simulink library "lateralFlightController"  (R2018b)
settings: Solver=VariableStepAuto  StartTime=0.0  StopTime=10.0  RelTol=1e-3
values from neighbouring files (symbols this model uses):
  kdRollMom = 5000*(pi/180)*MOI_X    [lateralFlight_ts.m]
  kdVelAng = 6*kpVelAng    (= 48)    [lateralFlight_ts.m]
  kpRollMom = 25000*(pi/180)*MOI_X    [lateralFlight_ts.m]
  kpVelAng = maxBank/(5*(pi/180))    (= 8)    [lateralFlight_ts.m]
  maxBank = 40*pi/180    (= 0.698131700798)    [lateralFlight_ts.m]
  tauRollMom = .01    (= 0.01)    [lateralFlight_ts.m]
  tauVelAng = .01    (= 0.01)    [lateralFlight_ts.m]
libraries: setpointToOutput_cl x2, filteredPIDController_ul x2, cartToSphere_ul x1, vrlib x1, schmehlTangentRotation_ul x1
settings Model: Creator=James Reed  LastModifiedBy=jldanie5

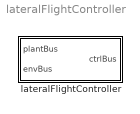
== system lateralFlightController ==
  lateralFlightController : Subsystem

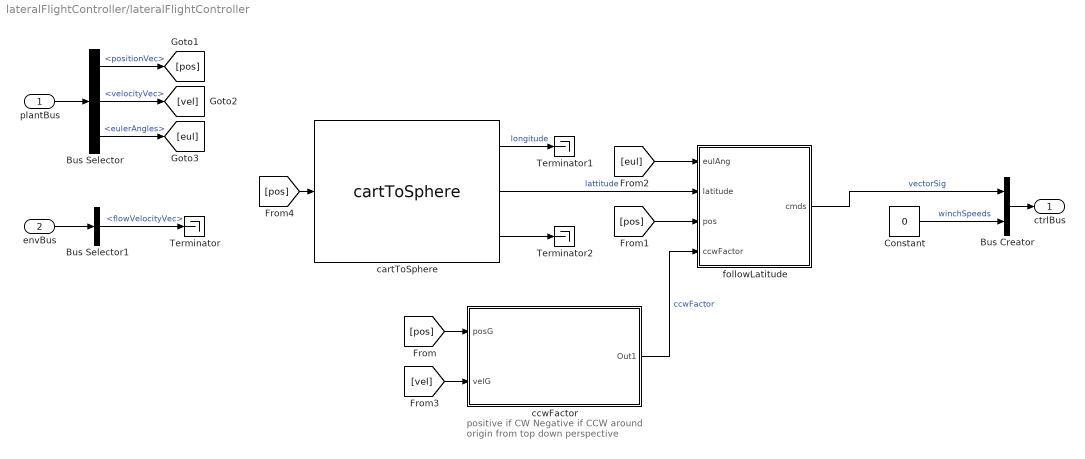
== system lateralFlightController/lateralFlightController ==
  note: positive if CW
      | Negative if CCW
      | around origin from top down perspective
  plantBus : Inport  OutDataTypeStr=Bus: plantBus
  envBus : Inport  Port=2  OutDataTypeStr=Bus: envBus
  Bus Creator : BusCreator  Inputs=2  OutDataTypeStr=Bus: ctrlBus
  Bus Selector : BusSelector  OutputSignals=positionVec,velocityVec,eulerAngles
  Bus Selector1 : BusSelector  OutputSignals=flowVelocityVec
  Constant : Constant  Value=0
  Terminator : Terminator
  Terminator1 : Terminator
  Terminator2 : Terminator
  cartToSphere : cartToSphere_ul/cartToSphere  SystemSampleTime=-1
  ccwFactor : Subsystem
  followLatitude : Subsystem  mask{kpVelAngMask=kpVelAng, kdVelAngMask=kdVelAng, tauVelAngMask=tauVelAng, kpLMask=kpRollMom, kdLMask=kdRollMom, tauLMask=tauRollMom, maxBankMask=maxBank, latDes=pi/4}
      mask prompts: kpVelAngMask "Proportional Gain Velocity Angle"; kdVelAngMask "Derivative Gain Velocity Angle"; tauVelAngMask "Tau Velocity Angle"; kpLMask "Proportional Gain TanRoll"; kdLMask "Derivative Gain Tanroll"; tauLMask "Tau Roll Moment"; maxBankMask "Max Bank Angle"; latDes "Desired Latitude"
  ctrlBus : Outport  OutDataTypeStr=Bus: ctrlBus
  wires:
  Bus Selector/3 -> [eul]  "<eulerAngles>"
  Bus Selector/1 -> [pos]  "<positionVec>"
  Bus Selector1/1 -> Terminator/1  "<flowVelocityVec>"
  Bus Selector/2 -> [vel]  "<velocityVec>"
  plantBus/1 -> Bus Selector/1
  envBus/1 -> Bus Selector1/1
  Bus Creator/1 -> ctrlBus/1
  followLatitude/1(cmds) -> Bus Creator/1  "vectorSig"
  Constant/1 -> Bus Creator/2  "winchSpeeds"
  [eul] -> followLatitude/1(eulAng)
  [pos] -> cartToSphere/1
  cartToSphere/1 -> Terminator1/1  "longitude"
  cartToSphere/3 -> Terminator2/1
  cartToSphere/2 -> followLatitude/2("latitude ")  "lattitude"
  [pos] -> followLatitude/3("pos ")
  [pos] -> ccwFactor/1(posG)
  [vel] -> ccwFactor/2(velG)
  ccwFactor/1(Out1) -> followLatitude/4(ccwFactor)  "ccwFactor"

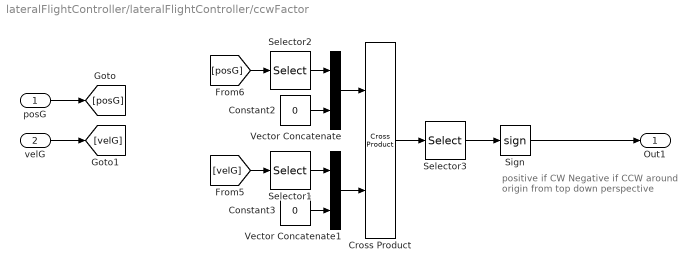
== system lateralFlightController/lateralFlightController/ccwFactor ==
  note: positive if CW
      | Negative if CCW
      | around origin from top down perspective
  posG : Inport
  velG : Inport  Port=2
  Constant2 : Constant  Value=0
  Constant3 : Constant  Value=0
  Cross Product : vrlib/Utilities/Cross Product
      settings: SourceProductBaseCode=VR
  Selector1 : Selector  InputPortWidth=3  IndexOptions=Index vector (dialog)  Indices=[1 2]  OutputSizes=1
  Selector2 : Selector  InputPortWidth=3  IndexOptions=Index vector (dialog)  Indices=[1 2]  OutputSizes=1
  Selector3 : Selector  InputPortWidth=3  IndexOptions=Index vector (dialog)  Indices=3  OutputSizes=1
  Sign : Signum
  Vector Concatenate : Concatenate
  Vector Concatenate1 : Concatenate
  Out1 : Outport
  wires:
  Sign/1 -> Out1/1
  Vector Concatenate1/1 -> Cross Product/2
  Vector Concatenate/1 -> Cross Product/1
  [posG] -> Selector2/1
  Selector1/1 -> Vector Concatenate1/1
  [velG] -> Selector1/1
  Selector2/1 -> Vector Concatenate/1
  Constant2/1 -> Vector Concatenate/2
  Constant3/1 -> Vector Concatenate1/2
  Selector3/1 -> Sign/1
  Cross Product/1 -> Selector3/1
  posG/1 -> [posG]
  velG/1 -> [velG]

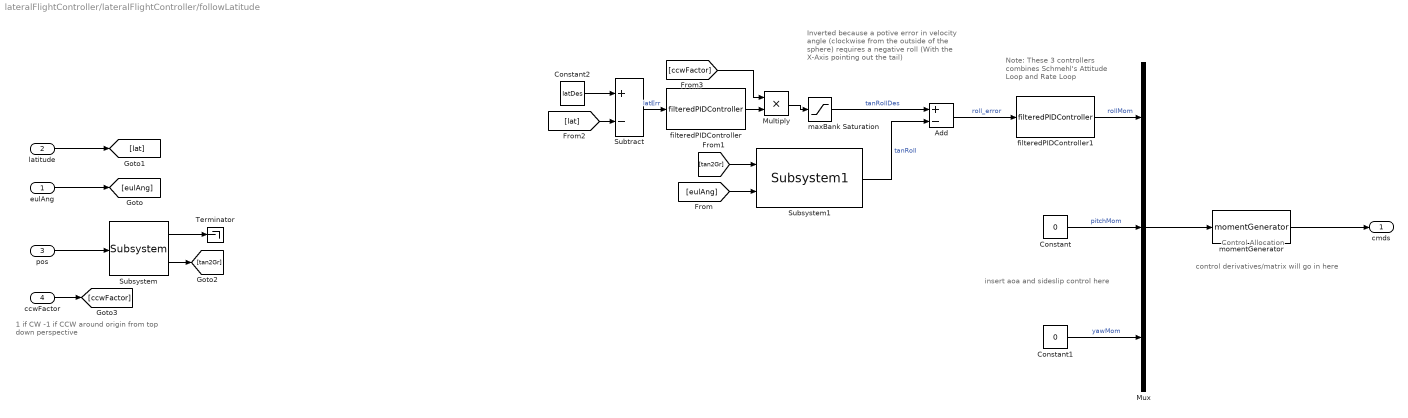
== system lateralFlightController/lateralFlightController/followLatitude ==
  note: control derivatives/matrix will go in here
  note: insert aoa and sideslip control here
  note: Control Allocation
  note: Inverted because a potive error
      | in velocity angle (clockwise from the
      | outside of the sphere) requires a negative
      | roll (With the X-Axis pointing out the tail)
  note: Note: These 3 controllers
      | combines Schmehl's Attitude
      | Loop and Rate Loop
  note: 1 if CW
      | -1 if CCW
      | around origin from top down perspective
  eulAng : Inport
  "latitude " : Inport  Port=2
  "pos " : Inport  Port=3
  ccwFactor : Inport  Port=4
  Add : Sum  Inputs=+-
  Constant : Constant  Value=0
  Constant1 : Constant  Value=0
  Constant2 : Constant  Value=latDes
  Multiply : Product
  Mux : Mux  Inputs=3
  Subsystem : schmehlTangentRotation_ul/Subsystem  SystemSampleTime=-1
  Subsystem1 : setpointToOutput_cl/Subsystem/Subsystem1  SystemSampleTime=-1
  Subtract : Sum  Inputs=+-
  Terminator : Terminator
  filteredPIDController : filteredPIDController_ul/filteredPIDController  kp=kpVelAngMask  ki=0  kd=kdVelAngMask  Value=tauVelAngMask
  filteredPIDController1 : filteredPIDController_ul/filteredPIDController  kp=kpLMask  ki=0  kd=kdLMask  Value=tauLMask
  maxBank Saturation : Saturate  UpperLimit=maxBankMask  LowerLimit=-maxBankMask
  momentGenerator : setpointToOutput_cl/Subsystem/momentGenerator  SystemSampleTime=-1
  cmds : Outport
  wires:
  [tan2Gr] -> Subsystem1/1
  Constant1/1 -> Mux/3  "yawMom"
  Add/1 -> filteredPIDController1/1  "roll_error"
  Multiply/1 -> maxBank Saturation/1
  Subsystem1/1 -> Add/2  "tanRoll"
  eulAng/1 -> [eulAng]
  filteredPIDController/1 -> Multiply/2
  [eulAng] -> Subsystem1/2
  Constant/1 -> Mux/2  "pitchMom"
  maxBank Saturation/1 -> Add/1  "tanRollDes"
  Mux/1 -> momentGenerator/1
  momentGenerator/1 -> cmds/1
  "latitude "/1 -> [lat]
  [lat] -> Subtract/2
  Constant2/1 -> Subtract/1
  Subtract/1 -> filteredPIDController/1  "latErr"
  "pos "/1 -> Subsystem/1
  Subsystem/2 -> [tan2Gr]
  Subsystem/1 -> Terminator/1
  filteredPIDController1/1 -> Mux/1  "rollMom"
  ccwFactor/1 -> [ccwFactor]
  [ccwFactor] -> Multiply/1
